simulink model "ProblemB"  (R2018a)
settings: Solver=VariableStepAuto  StartTime=0.0  StopTime=10.0  RelTol=1e-3
values from neighbouring files (symbols this model uses):
  Bm = 6.04e-6    (= 6.04e-06)    [pm_par.m]    (also in series_par.m)
  J = 1    [dc_par.m]    (also in pm_par.m = 2.12e-06; series_par.m = 2.12e-06)
  Laf = 1.8    [dc_par.m]    (also in series_par.m = 0.0395)
  Ra = 0.6    [dc_par.m]    (also in pm_par.m = 7; series_par.m = 6)
  Rf = 240    [dc_par.m]    (also in series_par.m = 1)
  Tf = Lf/Rf    (= 0.5)    [dc_par.m]
  Tm = 29    [dc_par.m]    (also in pm_par.m = 0.00353; series_par.m = 0.00353)
  Va = 240    [dc_par.m]    (also in pm_par.m = 6; series_par.m = 6)
settings Model: Creator=Jasper  LastModifiedBy=Jasper

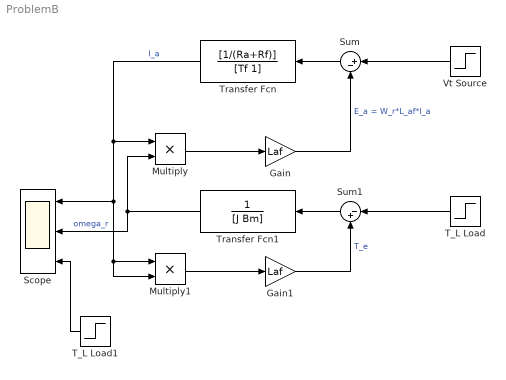
== system ProblemB ==
  Gain : Gain  Gain=Laf
  Gain1 : Gain  Gain=Laf
  Multiply : Product
  Multiply1 : Product
  Scope : Scope  NumInputPorts=3
  Sum : Sum  Inputs=|+-
  Sum1 : Sum  Inputs=|-+
  T_L Load : Step  Time=4  After=Tm  SampleTime=0
  T_L Load1 : Step  Time=4  After=Tm  SampleTime=0
  Transfer Fcn : TransferFcn  Numerator=[1/(Ra+Rf)]  Denominator=[Tf 1]
  Transfer Fcn1 : TransferFcn  Denominator=[J Bm]
  Vt Source : Step  Time=0  Before=Va  After=Va  SampleTime=0
  wires:
  Gain/1 -> Sum/2  "E_a = W_r*L_af*I_a"
  Multiply/1 -> Gain/1
  Vt Source/1 -> Sum/1
  Sum/1 -> Transfer Fcn/1
  Transfer Fcn/1 -> Multiply1/2, Multiply1/1, Scope/1, Multiply/1  "I_a"
  Transfer Fcn1/1 -> Scope/2, Multiply/2  "omega_r"
  Sum1/1 -> Transfer Fcn1/1
  Multiply1/1 -> Gain1/1
  Gain1/1 -> Sum1/2  "T_e"
  T_L Load/1 -> Sum1/1
  T_L Load1/1 -> Scope/3
